simulink library "ammclib_bam_s32k11x"  (Simulink 9.0)
settings: Solver=ode45  StartTime=0.0  StopTime=10.0  RelTol=1e-3
undefined symbols (not defined in the file): f16A1, f16A2, f16B0, f16B1, f16B2, f16C1, f16CC1, f16CC1sc, f16CC1sc_D, f16CC1sc_Q, f16CC1scD, f16CC1scQ, f16CC2, f16CC2sc, f16CC2sc_D, f16CC2sc_Q, f16CC2scD, f16CC2scQ, f16DerivGain, f16EGain, f16FiltCoef, f16HystOff, f16HystOn, f16IGain, f16IntegGain, f16IntegGainFW, f16IntegGainQ, f16Kd, f16Kq, f16Limit, f16LowerLim, f16LowerLimit_D, f16LowerLimit_Q, f16ModIndex, f16OutValOff, f16OutValOn, f16PropGain, f16PropGainFW, f16PropGainQ, f16RampDown, f16RampUp, f16UGain, f16UpperLim, f16UpperLimit, f16UpperLimit_D, f16UpperLimit_Q, f16WIGain, f32A1, f32A2, f32B0, f32B1, f32B2, f32C1, f32CC1, f32CC1sc, f32CC1sc_D, f32CC1sc_Q, f32CC1scD, f32CC1scQ, f32CC2 ... (+71)
(part 7 of 7)

== system ammclib_bam_s32k11x/MLIB/bam_f32/MLIB_SubSat_F32 ==
  note: ---------------------------------------------------------------------------------------------------------------------------------------------------------------------------------------------------
  f32In1 : Inport
  f32In2 : Inport  Port=2
  MLIB_SubSat_SF : S-Function  FunctionName=MLIB_SubSat_SF_F32  SFunctionDeploymentMode=off  EnableBusSupport=off
  copyright : Subsystem
      mask Display:
      | text(10,90,'FILE:');text(10,75,'DESRIPTION:')
      | text(10,60,'COPYRIGHT:')
      | text(10,45,'VERSION:')
      | text(10,30,'DATE:')
  copyright2 : Subsystem
      mask Display:
      | text(10,90,'MLIB_SubSat_BAM_F32.mdl');text(10,75,'Saturated sum of two input values.');text(10,60,'NXP')
      | text(10,45,'0.1');text(10,30,'20-Jan-2012');
  logo : Subsystem
      mask Display: image(imread('logo.jpg'))
  f32Out : Outport
  wires:
  MLIB_SubSat_SF/1 -> f32Out/1
  f32In2/1 -> MLIB_SubSat_SF/2
  f32In1/1 -> MLIB_SubSat_SF/1

== system ammclib_bam_s32k11x/MLIB/bam_f32/MLIB_Sub_F32 ==
  note: ---------------------------------------------------------------------------------------------------------------------------------------------------------------------------------------------------
  f32In1 : Inport
  f32In2 : Inport  Port=2
  MLIB_Sub_SF : S-Function  FunctionName=MLIB_Sub_SF_F32  SFunctionDeploymentMode=off  EnableBusSupport=off
  copyright : Subsystem
      mask Display:
      | text(10,90,'FILE:');text(10,75,'DESRIPTION:')
      | text(10,60,'COPYRIGHT:')
      | text(10,45,'VERSION:')
      | text(10,30,'DATE:')
  copyright2 : Subsystem
      mask Display:
      | text(10,90,'MLIB_Sub_BAM_F32.mdl');text(10,75,'Sum of two input values.');text(10,60,'NXP')
      | text(10,45,'0.1');text(10,30,'18-Jul-2011');
  logo : Subsystem
      mask Display: image(imread('logo.jpg'))
  f32Out : Outport
  wires:
  MLIB_Sub_SF/1 -> f32Out/1
  f32In2/1 -> MLIB_Sub_SF/2
  f32In1/1 -> MLIB_Sub_SF/1

== system ammclib_bam_s32k11x/MLIB/bam_f32/MLIB_VMac_F32 ==
  note: ---------------------------------------------------------------------------------------------------------------------------------------------------------------------------------------------------
  f32In1 : Inport
  f32In2 : Inport  Port=2
  f32In3 : Inport  Port=3
  f32In4 : Inport  Port=4
  MLIB_VMac_SF : S-Function  FunctionName=MLIB_VMac_SF_F32  SFunctionDeploymentMode=off  EnableBusSupport=off
  copyright : Subsystem
      mask Display:
      | text(10,90,'FILE:');text(10,75,'DESRIPTION:')
      | text(10,60,'COPYRIGHT:')
      | text(10,45,'VERSION:')
      | text(10,30,'DATE:')
  copyright2 : Subsystem
      mask Display:
      | text(10,90,'MLIB_VMac_BAM_F32.mdl');text(10,75,'Vector multiply accumulate.');text(10,60,'Freescale')
      | text(10,45,'0.1');text(10,30,'25-Aug-2011');
  logo : Subsystem
      mask Display: image(imread('logo.jpg'))
  f32Out : Outport
  wires:
  MLIB_VMac_SF/1 -> f32Out/1
  f32In4/1 -> MLIB_VMac_SF/4
  f32In3/1 -> MLIB_VMac_SF/3
  f32In2/1 -> MLIB_VMac_SF/2
  f32In1/1 -> MLIB_VMac_SF/1

== system ammclib_bam_s32k11x/MLIB/bam_f32f16f16/MLIB_MacSat_F32F16F16 ==
  note: ---------------------------------------------------------------------------------------------------------------------------------------------------------------------------------------------------
  f32In1 : Inport
  f16In2 : Inport  Port=2
  f16In3 : Inport  Port=3
  MLIB_MacSat_SF : S-Function  FunctionName=MLIB_MacSat_SF_F32F16F16  SFunctionDeploymentMode=off  EnableBusSupport=off
  copyright : Subsystem
      mask Display:
      | text(10,90,'FILE:');text(10,75,'DESRIPTION:')
      | text(10,60,'COPYRIGHT:')
      | text(10,45,'VERSION:')
      | text(10,30,'DATE:')
  copyright2 : Subsystem
      mask Display:
      | text(10,90,'MLIB_MacSat_BAM_F32F16F16.mdl');text(10,75,'Multiplication of second and third input value and adding of first input value, staturated if necessary.');text(10,60,'NXP')
      | text(10,45,'0.1');text(10,30,'22-Aug-2011');
  logo : Subsystem
      mask Display: image(imread('logo.jpg'))
  f32Out : Outport
  wires:
  MLIB_MacSat_SF/1 -> f32Out/1
  f16In3/1 -> MLIB_MacSat_SF/3
  f16In2/1 -> MLIB_MacSat_SF/2
  f32In1/1 -> MLIB_MacSat_SF/1

== system ammclib_bam_s32k11x/MLIB/bam_f32f16f16/MLIB_Mac_F32F16F16 ==
  note: ---------------------------------------------------------------------------------------------------------------------------------------------------------------------------------------------------
  f32In1 : Inport
  f16In2 : Inport  Port=2
  f16In3 : Inport  Port=3
  MLIB_Mac_SF : S-Function  FunctionName=MLIB_Mac_SF_F32F16F16  SFunctionDeploymentMode=off  EnableBusSupport=off
  copyright : Subsystem
      mask Display:
      | text(10,90,'FILE:');text(10,75,'DESRIPTION:')
      | text(10,60,'COPYRIGHT:')
      | text(10,45,'VERSION:')
      | text(10,30,'DATE:')
  copyright2 : Subsystem
      mask Display:
      | text(10,90,'MLIB_Mac_BAM_F32F16F16.mdl');text(10,75,'Sum of two input values.');text(10,60,'Freescale')
      | text(10,45,'0.1');text(10,30,'18-Jul-2011');
  logo : Subsystem
      mask Display: image(imread('logo.jpg'))
  f32Out : Outport
  wires:
  MLIB_Mac_SF/1 -> f32Out/1
  f16In3/1 -> MLIB_Mac_SF/3
  f16In2/1 -> MLIB_Mac_SF/2
  f32In1/1 -> MLIB_Mac_SF/1

== system ammclib_bam_s32k11x/MLIB/bam_f32f16f16/MLIB_Mnac_F32F16F16 ==
  note: ---------------------------------------------------------------------------------------------------------------------------------------------------------------------------------------------------
  f32In1 : Inport
  f16In2 : Inport  Port=2
  f16In3 : Inport  Port=3
  MLIB_Mnac_SF : S-Function  FunctionName=MLIB_Mnac_SF_F32F16F16  SFunctionDeploymentMode=off  EnableBusSupport=off
  copyright : Subsystem
      mask Display:
      | text(10,90,'FILE:');text(10,75,'DESRIPTION:')
      | text(10,60,'COPYRIGHT:')
      | text(10,45,'VERSION:')
      | text(10,30,'DATE:')
  copyright2 : Subsystem
      mask Display:
      | text(10,90,'MLIB_Mnac_BAM_F32F16F16.mdl');text(10,75,'Multiply-negative-accumulate.');text(10,60,'NXP')
      | text(10,45,'1.0');text(10,30,'27-Mar-2015');
  logo : Subsystem
      mask Display: image(imread('logo.jpg'))
  f32Out : Outport
  wires:
  MLIB_Mnac_SF/1 -> f32Out/1
  f16In3/1 -> MLIB_Mnac_SF/3
  f16In2/1 -> MLIB_Mnac_SF/2
  f32In1/1 -> MLIB_Mnac_SF/1

== system ammclib_bam_s32k11x/MLIB/bam_f32f16f16/MLIB_Msu_F32F16F16 ==
  note: ---------------------------------------------------------------------------------------------------------------------------------------------------------------------------------------------------
  f32In1 : Inport
  f16In2 : Inport  Port=2
  f16In3 : Inport  Port=3
  MLIB_Msu_SF : S-Function  FunctionName=MLIB_Msu_SF_F32F16F16  SFunctionDeploymentMode=off  EnableBusSupport=off
  copyright : Subsystem
      mask Display:
      | text(10,90,'FILE:');text(10,75,'DESRIPTION:')
      | text(10,60,'COPYRIGHT:')
      | text(10,45,'VERSION:')
      | text(10,30,'DATE:')
  copyright2 : Subsystem
      mask Display:
      | text(10,90,'MLIB_Msu_BAM_F32F16F16.mdl');text(10,75,'Multiply-subtract-from.');text(10,60,'Freescale')
      | text(10,45,'1.0');text(10,30,'27-Mar-2015');
  logo : Subsystem
      mask Display: image(imread('logo.jpg'))
  f32Out : Outport
  wires:
  MLIB_Msu_SF/1 -> f32Out/1
  f16In3/1 -> MLIB_Msu_SF/3
  f16In2/1 -> MLIB_Msu_SF/2
  f32In1/1 -> MLIB_Msu_SF/1

== system ammclib_bam_s32k11x/MLIB/bam_f32f16f16/MLIB_MulSat_F32F16F16 ==
  note: ---------------------------------------------------------------------------------------------------------------------------------------------------------------------------------------------------
  f16In1 : Inport
  f16In2 : Inport  Port=2
  MLIB_MulSat_SF : S-Function  FunctionName=MLIB_MulSat_SF_F32F16F16  SFunctionDeploymentMode=off  EnableBusSupport=off
  copyright : Subsystem
      mask Display:
      | text(10,90,'FILE:');text(10,75,'DESRIPTION:')
      | text(10,60,'COPYRIGHT:')
      | text(10,45,'VERSION:')
      | text(10,30,'DATE:')
  copyright2 : Subsystem
      mask Display:
      | text(10,90,'MLIB_MulSat_BAM_F32F16F16.mdl');text(10,75,'Saturated sum of two input values.');text(10,60,'NXP')
      | text(10,45,'0.1');text(10,30,'01-Aug-2011');
  logo : Subsystem
      mask Display: image(imread('logo.jpg'))
  f32Out : Outport
  wires:
  MLIB_MulSat_SF/1 -> f32Out/1
  f16In2/1 -> MLIB_MulSat_SF/2
  f16In1/1 -> MLIB_MulSat_SF/1

== system ammclib_bam_s32k11x/MLIB/bam_f32f16f16/MLIB_Mul_F32F16F16 ==
  note: ---------------------------------------------------------------------------------------------------------------------------------------------------------------------------------------------------
  f16In1 : Inport
  f16In2 : Inport  Port=2
  MLIB_Mul_SF : S-Function  FunctionName=MLIB_Mul_SF_F32F16F16  SFunctionDeploymentMode=off  EnableBusSupport=off
  copyright : Subsystem
      mask Display:
      | text(10,90,'FILE:');text(10,75,'DESRIPTION:')
      | text(10,60,'COPYRIGHT:')
      | text(10,45,'VERSION:')
      | text(10,30,'DATE:')
  copyright2 : Subsystem
      mask Display:
      | text(10,90,'MLIB_Mul_BAM_F32F16F16.mdl');text(10,75,'Sum of two input values.');text(10,60,'Freescale')
      | text(10,45,'0.1');text(10,30,'26-Jul-2011');
  logo : Subsystem
      mask Display: image(imread('logo.jpg'))
  f32Out : Outport
  wires:
  MLIB_Mul_SF/1 -> f32Out/1
  f16In2/1 -> MLIB_Mul_SF/2
  f16In1/1 -> MLIB_Mul_SF/1

== system ammclib_bam_s32k11x/MLIB/bam_f32f16f16/MLIB_VMac_F32F16F16 ==
  note: ---------------------------------------------------------------------------------------------------------------------------------------------------------------------------------------------------
  f16In1 : Inport
  f16In2 : Inport  Port=2
  f16In3 : Inport  Port=3
  f16In4 : Inport  Port=4
  MLIB_VMac_SF : S-Function  FunctionName=MLIB_VMac_SF_F32F16F16  SFunctionDeploymentMode=off  EnableBusSupport=off
  copyright : Subsystem
      mask Display:
      | text(10,90,'FILE:');text(10,75,'DESRIPTION:')
      | text(10,60,'COPYRIGHT:')
      | text(10,45,'VERSION:')
      | text(10,30,'DATE:')
  copyright2 : Subsystem
      mask Display:
      | text(10,90,'MLIB_VMac_BAM_F32F16F16.mdl');text(10,75,'Vector multiply accumulate.');text(10,60,'Freescale')
      | text(10,45,'0.1');text(10,30,'25-Aug-2011');
  logo : Subsystem
      mask Display: image(imread('logo.jpg'))
  f32Out : Outport
  wires:
  MLIB_VMac_SF/1 -> f32Out/1
  f16In4/1 -> MLIB_VMac_SF/4
  f16In3/1 -> MLIB_VMac_SF/3
  f16In2/1 -> MLIB_VMac_SF/2
  f16In1/1 -> MLIB_VMac_SF/1

== system ammclib_bam_s32k11x/AMCLIB/bam_f16/AMCLIB_BemfObsrvDQ_F16/copyright ==

== system ammclib_bam_s32k11x/AMCLIB/bam_f16/AMCLIB_BemfObsrvDQ_F16/copyright2 ==

== system ammclib_bam_s32k11x/AMCLIB/bam_f16/AMCLIB_BemfObsrvDQ_F16/logo ==

== system ammclib_bam_s32k11x/AMCLIB/bam_f16/AMCLIB_CurrentLoop_F16/copyright ==

== system ammclib_bam_s32k11x/AMCLIB/bam_f16/AMCLIB_CurrentLoop_F16/copyright2 ==

== system ammclib_bam_s32k11x/AMCLIB/bam_f16/AMCLIB_CurrentLoop_F16/logo ==

== system ammclib_bam_s32k11x/AMCLIB/bam_f16/AMCLIB_FWSpeedLoop_F16/copyright ==

== system ammclib_bam_s32k11x/AMCLIB/bam_f16/AMCLIB_FWSpeedLoop_F16/copyright2 ==

== system ammclib_bam_s32k11x/AMCLIB/bam_f16/AMCLIB_FWSpeedLoop_F16/logo ==

== system ammclib_bam_s32k11x/AMCLIB/bam_f16/AMCLIB_FW_F16/copyright ==

== system ammclib_bam_s32k11x/AMCLIB/bam_f16/AMCLIB_FW_F16/copyright2 ==

== system ammclib_bam_s32k11x/AMCLIB/bam_f16/AMCLIB_FW_F16/logo ==

== system ammclib_bam_s32k11x/AMCLIB/bam_f16/AMCLIB_SpeedLoop_F16/copyright ==

== system ammclib_bam_s32k11x/AMCLIB/bam_f16/AMCLIB_SpeedLoop_F16/copyright2 ==

== system ammclib_bam_s32k11x/AMCLIB/bam_f16/AMCLIB_SpeedLoop_F16/logo ==

== system ammclib_bam_s32k11x/AMCLIB/bam_f16/AMCLIB_TrackObsrv_F16/copyright ==

== system ammclib_bam_s32k11x/AMCLIB/bam_f16/AMCLIB_TrackObsrv_F16/copyright2 ==

== system ammclib_bam_s32k11x/AMCLIB/bam_f16/AMCLIB_TrackObsrv_F16/logo ==

== system ammclib_bam_s32k11x/AMCLIB/bam_f32/AMCLIB_BemfObsrvDQ_F32/copyright ==

== system ammclib_bam_s32k11x/AMCLIB/bam_f32/AMCLIB_BemfObsrvDQ_F32/copyright2 ==

== system ammclib_bam_s32k11x/AMCLIB/bam_f32/AMCLIB_BemfObsrvDQ_F32/logo ==

== system ammclib_bam_s32k11x/AMCLIB/bam_f32/AMCLIB_CurrentLoop_F32/copyright ==

== system ammclib_bam_s32k11x/AMCLIB/bam_f32/AMCLIB_CurrentLoop_F32/copyright2 ==

== system ammclib_bam_s32k11x/AMCLIB/bam_f32/AMCLIB_CurrentLoop_F32/logo ==

== system ammclib_bam_s32k11x/AMCLIB/bam_f32/AMCLIB_FWSpeedLoop_F32/copyright ==

== system ammclib_bam_s32k11x/AMCLIB/bam_f32/AMCLIB_FWSpeedLoop_F32/copyright2 ==

== system ammclib_bam_s32k11x/AMCLIB/bam_f32/AMCLIB_FWSpeedLoop_F32/logo ==

== system ammclib_bam_s32k11x/AMCLIB/bam_f32/AMCLIB_FW_F32/copyright ==

== system ammclib_bam_s32k11x/AMCLIB/bam_f32/AMCLIB_FW_F32/copyright2 ==

== system ammclib_bam_s32k11x/AMCLIB/bam_f32/AMCLIB_FW_F32/logo ==

== system ammclib_bam_s32k11x/AMCLIB/bam_f32/AMCLIB_SpeedLoop_F32/copyright ==

== system ammclib_bam_s32k11x/AMCLIB/bam_f32/AMCLIB_SpeedLoop_F32/copyright2 ==

== system ammclib_bam_s32k11x/AMCLIB/bam_f32/AMCLIB_SpeedLoop_F32/logo ==

== system ammclib_bam_s32k11x/AMCLIB/bam_f32/AMCLIB_TrackObsrv_F32/copyright ==

== system ammclib_bam_s32k11x/AMCLIB/bam_f32/AMCLIB_TrackObsrv_F32/copyright2 ==

== system ammclib_bam_s32k11x/AMCLIB/bam_f32/AMCLIB_TrackObsrv_F32/logo ==

== system ammclib_bam_s32k11x/GDFLIB/bam_f16/GDFLIB_FilterFIR_F16/copyright ==

== system ammclib_bam_s32k11x/GDFLIB/bam_f16/GDFLIB_FilterFIR_F16/copyright2 ==

== system ammclib_bam_s32k11x/GDFLIB/bam_f16/GDFLIB_FilterFIR_F16/logo ==

== system ammclib_bam_s32k11x/GDFLIB/bam_f16/GDFLIB_FilterIIR1_F16/copyright ==

== system ammclib_bam_s32k11x/GDFLIB/bam_f16/GDFLIB_FilterIIR1_F16/copyright2 ==

== system ammclib_bam_s32k11x/GDFLIB/bam_f16/GDFLIB_FilterIIR1_F16/logo ==

== system ammclib_bam_s32k11x/GDFLIB/bam_f16/GDFLIB_FilterIIR2_F16/copyright ==

== system ammclib_bam_s32k11x/GDFLIB/bam_f16/GDFLIB_FilterIIR2_F16/copyright2 ==

== system ammclib_bam_s32k11x/GDFLIB/bam_f16/GDFLIB_FilterIIR2_F16/logo ==

== system ammclib_bam_s32k11x/GDFLIB/bam_f16/GDFLIB_FilterMA_F16/copyright ==

== system ammclib_bam_s32k11x/GDFLIB/bam_f16/GDFLIB_FilterMA_F16/copyright2 ==

== system ammclib_bam_s32k11x/GDFLIB/bam_f16/GDFLIB_FilterMA_F16/logo ==

== system ammclib_bam_s32k11x/GDFLIB/bam_f32/GDFLIB_FilterFIR_F32/copyright ==

== system ammclib_bam_s32k11x/GDFLIB/bam_f32/GDFLIB_FilterFIR_F32/copyright2 ==

== system ammclib_bam_s32k11x/GDFLIB/bam_f32/GDFLIB_FilterFIR_F32/logo ==

== system ammclib_bam_s32k11x/GDFLIB/bam_f32/GDFLIB_FilterIIR1_F32/copyright ==

== system ammclib_bam_s32k11x/GDFLIB/bam_f32/GDFLIB_FilterIIR1_F32/copyright2 ==

== system ammclib_bam_s32k11x/GDFLIB/bam_f32/GDFLIB_FilterIIR1_F32/logo ==

== system ammclib_bam_s32k11x/GDFLIB/bam_f32/GDFLIB_FilterIIR2_F32/copyright ==

== system ammclib_bam_s32k11x/GDFLIB/bam_f32/GDFLIB_FilterIIR2_F32/copyright2 ==

== system ammclib_bam_s32k11x/GDFLIB/bam_f32/GDFLIB_FilterIIR2_F32/logo ==

== system ammclib_bam_s32k11x/GDFLIB/bam_f32/GDFLIB_FilterMA_F32/copyright ==

== system ammclib_bam_s32k11x/GDFLIB/bam_f32/GDFLIB_FilterMA_F32/copyright2 ==

== system ammclib_bam_s32k11x/GDFLIB/bam_f32/GDFLIB_FilterMA_F32/logo ==

== system ammclib_bam_s32k11x/GFLIB/bam_f16/GFLIB_Acos_F16/copyright ==

== system ammclib_bam_s32k11x/GFLIB/bam_f16/GFLIB_Acos_F16/copyright2 ==

== system ammclib_bam_s32k11x/GFLIB/bam_f16/GFLIB_Acos_F16/logo ==

== system ammclib_bam_s32k11x/GFLIB/bam_f16/GFLIB_Asin_F16/copyright ==

== system ammclib_bam_s32k11x/GFLIB/bam_f16/GFLIB_Asin_F16/copyright2 ==

== system ammclib_bam_s32k11x/GFLIB/bam_f16/GFLIB_Asin_F16/logo ==

== system ammclib_bam_s32k11x/GFLIB/bam_f16/GFLIB_AtanYXShifted_F16/copyright ==

== system ammclib_bam_s32k11x/GFLIB/bam_f16/GFLIB_AtanYXShifted_F16/copyright2 ==

== system ammclib_bam_s32k11x/GFLIB/bam_f16/GFLIB_AtanYXShifted_F16/logo ==

== system ammclib_bam_s32k11x/GFLIB/bam_f16/GFLIB_AtanYX_F16/copyright ==

== system ammclib_bam_s32k11x/GFLIB/bam_f16/GFLIB_AtanYX_F16/copyright2 ==

== system ammclib_bam_s32k11x/GFLIB/bam_f16/GFLIB_AtanYX_F16/logo ==

== system ammclib_bam_s32k11x/GFLIB/bam_f16/GFLIB_Atan_F16/copyright ==

== system ammclib_bam_s32k11x/GFLIB/bam_f16/GFLIB_Atan_F16/copyright2 ==

== system ammclib_bam_s32k11x/GFLIB/bam_f16/GFLIB_Atan_F16/logo ==

== system ammclib_bam_s32k11x/GFLIB/bam_f16/GFLIB_ControllerPIDpAW_F16/copyright ==

== system ammclib_bam_s32k11x/GFLIB/bam_f16/GFLIB_ControllerPIDpAW_F16/copyright2 ==

== system ammclib_bam_s32k11x/GFLIB/bam_f16/GFLIB_ControllerPIDpAW_F16/logo ==

== system ammclib_bam_s32k11x/GFLIB/bam_f16/GFLIB_ControllerPIpAW_F16/copyright ==

== system ammclib_bam_s32k11x/GFLIB/bam_f16/GFLIB_ControllerPIpAW_F16/copyright2 ==

== system ammclib_bam_s32k11x/GFLIB/bam_f16/GFLIB_ControllerPIpAW_F16/logo ==

== system ammclib_bam_s32k11x/GFLIB/bam_f16/GFLIB_ControllerPIp_F16/copyright ==

== system ammclib_bam_s32k11x/GFLIB/bam_f16/GFLIB_ControllerPIp_F16/copyright2 ==

== system ammclib_bam_s32k11x/GFLIB/bam_f16/GFLIB_ControllerPIp_F16/logo ==

== system ammclib_bam_s32k11x/GFLIB/bam_f16/GFLIB_ControllerPIrAW_F16/copyright ==

== system ammclib_bam_s32k11x/GFLIB/bam_f16/GFLIB_ControllerPIrAW_F16/copyright2 ==

== system ammclib_bam_s32k11x/GFLIB/bam_f16/GFLIB_ControllerPIrAW_F16/logo ==

== system ammclib_bam_s32k11x/GFLIB/bam_f16/GFLIB_ControllerPIr_F16/copyright ==

== system ammclib_bam_s32k11x/GFLIB/bam_f16/GFLIB_ControllerPIr_F16/copyright2 ==

== system ammclib_bam_s32k11x/GFLIB/bam_f16/GFLIB_ControllerPIr_F16/logo ==

== system ammclib_bam_s32k11x/GFLIB/bam_f16/GFLIB_Cos_F16/copyright ==

== system ammclib_bam_s32k11x/GFLIB/bam_f16/GFLIB_Cos_F16/copyright2 ==

== system ammclib_bam_s32k11x/GFLIB/bam_f16/GFLIB_Cos_F16/logo ==

== system ammclib_bam_s32k11x/GFLIB/bam_f16/GFLIB_Hyst_F16/copyright ==

== system ammclib_bam_s32k11x/GFLIB/bam_f16/GFLIB_Hyst_F16/copyright2 ==

== system ammclib_bam_s32k11x/GFLIB/bam_f16/GFLIB_Hyst_F16/logo ==

== system ammclib_bam_s32k11x/GFLIB/bam_f16/GFLIB_IntegratorTR_F16/copyright ==

== system ammclib_bam_s32k11x/GFLIB/bam_f16/GFLIB_IntegratorTR_F16/copyright2 ==

== system ammclib_bam_s32k11x/GFLIB/bam_f16/GFLIB_IntegratorTR_F16/logo ==

== system ammclib_bam_s32k11x/GFLIB/bam_f16/GFLIB_Limit_F16/copyright ==

== system ammclib_bam_s32k11x/GFLIB/bam_f16/GFLIB_Limit_F16/copyright2 ==

== system ammclib_bam_s32k11x/GFLIB/bam_f16/GFLIB_Limit_F16/logo ==

== system ammclib_bam_s32k11x/GFLIB/bam_f16/GFLIB_LowerLimit_F16/copyright ==

== system ammclib_bam_s32k11x/GFLIB/bam_f16/GFLIB_LowerLimit_F16/copyright2 ==

== system ammclib_bam_s32k11x/GFLIB/bam_f16/GFLIB_LowerLimit_F16/logo ==

== system ammclib_bam_s32k11x/GFLIB/bam_f16/GFLIB_Lut1D_F16/copyright ==

== system ammclib_bam_s32k11x/GFLIB/bam_f16/GFLIB_Lut1D_F16/copyright2 ==

== system ammclib_bam_s32k11x/GFLIB/bam_f16/GFLIB_Lut1D_F16/logo ==

== system ammclib_bam_s32k11x/GFLIB/bam_f16/GFLIB_Lut2D_F16/copyright ==

== system ammclib_bam_s32k11x/GFLIB/bam_f16/GFLIB_Lut2D_F16/copyright2 ==

== system ammclib_bam_s32k11x/GFLIB/bam_f16/GFLIB_Lut2D_F16/logo ==

== system ammclib_bam_s32k11x/GFLIB/bam_f16/GFLIB_Ramp_F16/copyright ==

== system ammclib_bam_s32k11x/GFLIB/bam_f16/GFLIB_Ramp_F16/copyright2 ==

== system ammclib_bam_s32k11x/GFLIB/bam_f16/GFLIB_Ramp_F16/logo ==

== system ammclib_bam_s32k11x/GFLIB/bam_f16/GFLIB_Sign_F16/copyright ==

== system ammclib_bam_s32k11x/GFLIB/bam_f16/GFLIB_Sign_F16/copyright2 ==

== system ammclib_bam_s32k11x/GFLIB/bam_f16/GFLIB_Sign_F16/logo ==

== system ammclib_bam_s32k11x/GFLIB/bam_f16/GFLIB_SinCos_F16/copyright ==

== system ammclib_bam_s32k11x/GFLIB/bam_f16/GFLIB_SinCos_F16/copyright2 ==

== system ammclib_bam_s32k11x/GFLIB/bam_f16/GFLIB_SinCos_F16/logo ==

== system ammclib_bam_s32k11x/GFLIB/bam_f16/GFLIB_Sin_F16/copyright ==

== system ammclib_bam_s32k11x/GFLIB/bam_f16/GFLIB_Sin_F16/copyright2 ==

== system ammclib_bam_s32k11x/GFLIB/bam_f16/GFLIB_Sin_F16/logo ==

== system ammclib_bam_s32k11x/GFLIB/bam_f16/GFLIB_Sqrt_F16/copyright ==

== system ammclib_bam_s32k11x/GFLIB/bam_f16/GFLIB_Sqrt_F16/copyright2 ==

== system ammclib_bam_s32k11x/GFLIB/bam_f16/GFLIB_Sqrt_F16/logo ==

== system ammclib_bam_s32k11x/GFLIB/bam_f16/GFLIB_Tan_F16/copyright ==

== system ammclib_bam_s32k11x/GFLIB/bam_f16/GFLIB_Tan_F16/copyright2 ==

== system ammclib_bam_s32k11x/GFLIB/bam_f16/GFLIB_Tan_F16/logo ==

== system ammclib_bam_s32k11x/GFLIB/bam_f16/GFLIB_UpperLimit_F16/copyright ==

== system ammclib_bam_s32k11x/GFLIB/bam_f16/GFLIB_UpperLimit_F16/copyright2 ==

== system ammclib_bam_s32k11x/GFLIB/bam_f16/GFLIB_UpperLimit_F16/logo ==

== system ammclib_bam_s32k11x/GFLIB/bam_f16/GFLIB_VMin_F16/copyright ==

== system ammclib_bam_s32k11x/GFLIB/bam_f16/GFLIB_VMin_F16/copyright2 ==

== system ammclib_bam_s32k11x/GFLIB/bam_f16/GFLIB_VMin_F16/logo ==

== system ammclib_bam_s32k11x/GFLIB/bam_f16/GFLIB_VectorLimit_F16/copyright ==

== system ammclib_bam_s32k11x/GFLIB/bam_f16/GFLIB_VectorLimit_F16/copyright2 ==

== system ammclib_bam_s32k11x/GFLIB/bam_f16/GFLIB_VectorLimit_F16/logo ==

== system ammclib_bam_s32k11x/GFLIB/bam_f32/GFLIB_Acos_F32/copyright ==

== system ammclib_bam_s32k11x/GFLIB/bam_f32/GFLIB_Acos_F32/copyright2 ==

== system ammclib_bam_s32k11x/GFLIB/bam_f32/GFLIB_Acos_F32/logo ==

== system ammclib_bam_s32k11x/GFLIB/bam_f32/GFLIB_Asin_F32/copyright ==

== system ammclib_bam_s32k11x/GFLIB/bam_f32/GFLIB_Asin_F32/copyright2 ==

== system ammclib_bam_s32k11x/GFLIB/bam_f32/GFLIB_Asin_F32/logo ==

== system ammclib_bam_s32k11x/GFLIB/bam_f32/GFLIB_AtanYXShifted_F32/copyright ==

== system ammclib_bam_s32k11x/GFLIB/bam_f32/GFLIB_AtanYXShifted_F32/copyright2 ==

== system ammclib_bam_s32k11x/GFLIB/bam_f32/GFLIB_AtanYXShifted_F32/logo ==

== system ammclib_bam_s32k11x/GFLIB/bam_f32/GFLIB_AtanYX_F32/copyright ==

== system ammclib_bam_s32k11x/GFLIB/bam_f32/GFLIB_AtanYX_F32/copyright2 ==

== system ammclib_bam_s32k11x/GFLIB/bam_f32/GFLIB_AtanYX_F32/logo ==

== system ammclib_bam_s32k11x/GFLIB/bam_f32/GFLIB_Atan_F32/copyright ==

== system ammclib_bam_s32k11x/GFLIB/bam_f32/GFLIB_Atan_F32/copyright2 ==

== system ammclib_bam_s32k11x/GFLIB/bam_f32/GFLIB_Atan_F32/logo ==

== system ammclib_bam_s32k11x/GFLIB/bam_f32/GFLIB_ControllerPIDpAW_F32/copyright ==

== system ammclib_bam_s32k11x/GFLIB/bam_f32/GFLIB_ControllerPIDpAW_F32/copyright2 ==

== system ammclib_bam_s32k11x/GFLIB/bam_f32/GFLIB_ControllerPIDpAW_F32/logo ==

== system ammclib_bam_s32k11x/GFLIB/bam_f32/GFLIB_ControllerPIpAW_F32/copyright ==

== system ammclib_bam_s32k11x/GFLIB/bam_f32/GFLIB_ControllerPIpAW_F32/copyright2 ==

== system ammclib_bam_s32k11x/GFLIB/bam_f32/GFLIB_ControllerPIpAW_F32/logo ==

== system ammclib_bam_s32k11x/GFLIB/bam_f32/GFLIB_ControllerPIp_F32/copyright ==

== system ammclib_bam_s32k11x/GFLIB/bam_f32/GFLIB_ControllerPIp_F32/copyright2 ==

== system ammclib_bam_s32k11x/GFLIB/bam_f32/GFLIB_ControllerPIp_F32/logo ==

== system ammclib_bam_s32k11x/GFLIB/bam_f32/GFLIB_ControllerPIrAW_F32/copyright ==

== system ammclib_bam_s32k11x/GFLIB/bam_f32/GFLIB_ControllerPIrAW_F32/copyright2 ==

== system ammclib_bam_s32k11x/GFLIB/bam_f32/GFLIB_ControllerPIrAW_F32/logo ==

== system ammclib_bam_s32k11x/GFLIB/bam_f32/GFLIB_ControllerPIr_F32/copyright ==

== system ammclib_bam_s32k11x/GFLIB/bam_f32/GFLIB_ControllerPIr_F32/copyright2 ==

== system ammclib_bam_s32k11x/GFLIB/bam_f32/GFLIB_ControllerPIr_F32/logo ==

== system ammclib_bam_s32k11x/GFLIB/bam_f32/GFLIB_Cos_F32/copyright ==

== system ammclib_bam_s32k11x/GFLIB/bam_f32/GFLIB_Cos_F32/copyright2 ==

== system ammclib_bam_s32k11x/GFLIB/bam_f32/GFLIB_Cos_F32/logo ==

== system ammclib_bam_s32k11x/GFLIB/bam_f32/GFLIB_Hyst_F32/copyright ==

== system ammclib_bam_s32k11x/GFLIB/bam_f32/GFLIB_Hyst_F32/copyright2 ==

== system ammclib_bam_s32k11x/GFLIB/bam_f32/GFLIB_Hyst_F32/logo ==

== system ammclib_bam_s32k11x/GFLIB/bam_f32/GFLIB_IntegratorTR_F32/copyright ==

== system ammclib_bam_s32k11x/GFLIB/bam_f32/GFLIB_IntegratorTR_F32/copyright2 ==

== system ammclib_bam_s32k11x/GFLIB/bam_f32/GFLIB_IntegratorTR_F32/logo ==

== system ammclib_bam_s32k11x/GFLIB/bam_f32/GFLIB_Limit_F32/copyright ==

== system ammclib_bam_s32k11x/GFLIB/bam_f32/GFLIB_Limit_F32/copyright2 ==

== system ammclib_bam_s32k11x/GFLIB/bam_f32/GFLIB_Limit_F32/logo ==

== system ammclib_bam_s32k11x/GFLIB/bam_f32/GFLIB_LowerLimit_F32/copyright ==

== system ammclib_bam_s32k11x/GFLIB/bam_f32/GFLIB_LowerLimit_F32/copyright2 ==

== system ammclib_bam_s32k11x/GFLIB/bam_f32/GFLIB_LowerLimit_F32/logo ==

== system ammclib_bam_s32k11x/GFLIB/bam_f32/GFLIB_Lut1D_F32/copyright ==

== system ammclib_bam_s32k11x/GFLIB/bam_f32/GFLIB_Lut1D_F32/copyright2 ==

== system ammclib_bam_s32k11x/GFLIB/bam_f32/GFLIB_Lut1D_F32/logo ==

== system ammclib_bam_s32k11x/GFLIB/bam_f32/GFLIB_Lut2D_F32/copyright ==

== system ammclib_bam_s32k11x/GFLIB/bam_f32/GFLIB_Lut2D_F32/copyright2 ==

== system ammclib_bam_s32k11x/GFLIB/bam_f32/GFLIB_Lut2D_F32/logo ==

== system ammclib_bam_s32k11x/GFLIB/bam_f32/GFLIB_Ramp_F32/copyright ==

== system ammclib_bam_s32k11x/GFLIB/bam_f32/GFLIB_Ramp_F32/copyright2 ==

== system ammclib_bam_s32k11x/GFLIB/bam_f32/GFLIB_Ramp_F32/logo ==

== system ammclib_bam_s32k11x/GFLIB/bam_f32/GFLIB_Sign_F32/copyright ==

== system ammclib_bam_s32k11x/GFLIB/bam_f32/GFLIB_Sign_F32/copyright2 ==

== system ammclib_bam_s32k11x/GFLIB/bam_f32/GFLIB_Sign_F32/logo ==

== system ammclib_bam_s32k11x/GFLIB/bam_f32/GFLIB_SinCos_F32/copyright ==

== system ammclib_bam_s32k11x/GFLIB/bam_f32/GFLIB_SinCos_F32/copyright2 ==

== system ammclib_bam_s32k11x/GFLIB/bam_f32/GFLIB_SinCos_F32/logo ==

== system ammclib_bam_s32k11x/GFLIB/bam_f32/GFLIB_Sin_F32/copyright ==

== system ammclib_bam_s32k11x/GFLIB/bam_f32/GFLIB_Sin_F32/copyright2 ==

== system ammclib_bam_s32k11x/GFLIB/bam_f32/GFLIB_Sin_F32/logo ==

== system ammclib_bam_s32k11x/GFLIB/bam_f32/GFLIB_Sqrt_F32/copyright ==

== system ammclib_bam_s32k11x/GFLIB/bam_f32/GFLIB_Sqrt_F32/copyright2 ==

== system ammclib_bam_s32k11x/GFLIB/bam_f32/GFLIB_Sqrt_F32/logo ==

== system ammclib_bam_s32k11x/GFLIB/bam_f32/GFLIB_Tan_F32/copyright ==

== system ammclib_bam_s32k11x/GFLIB/bam_f32/GFLIB_Tan_F32/copyright2 ==

== system ammclib_bam_s32k11x/GFLIB/bam_f32/GFLIB_Tan_F32/logo ==

== system ammclib_bam_s32k11x/GFLIB/bam_f32/GFLIB_UpperLimit_F32/copyright ==

== system ammclib_bam_s32k11x/GFLIB/bam_f32/GFLIB_UpperLimit_F32/copyright2 ==

== system ammclib_bam_s32k11x/GFLIB/bam_f32/GFLIB_UpperLimit_F32/logo ==

== system ammclib_bam_s32k11x/GFLIB/bam_f32/GFLIB_VMin_F32/copyright ==

== system ammclib_bam_s32k11x/GFLIB/bam_f32/GFLIB_VMin_F32/copyright2 ==

== system ammclib_bam_s32k11x/GFLIB/bam_f32/GFLIB_VMin_F32/logo ==

== system ammclib_bam_s32k11x/GFLIB/bam_f32/GFLIB_VectorLimit_F32/copyright ==

== system ammclib_bam_s32k11x/GFLIB/bam_f32/GFLIB_VectorLimit_F32/copyright2 ==

== system ammclib_bam_s32k11x/GFLIB/bam_f32/GFLIB_VectorLimit_F32/logo ==

== system ammclib_bam_s32k11x/GMCLIB/bam_f16/GMCLIB_ClarkInv_F16/copyright ==

== system ammclib_bam_s32k11x/GMCLIB/bam_f16/GMCLIB_ClarkInv_F16/copyright2 ==

== system ammclib_bam_s32k11x/GMCLIB/bam_f16/GMCLIB_ClarkInv_F16/logo ==

== system ammclib_bam_s32k11x/GMCLIB/bam_f16/GMCLIB_Clark_F16/copyright ==

== system ammclib_bam_s32k11x/GMCLIB/bam_f16/GMCLIB_Clark_F16/copyright2 ==

== system ammclib_bam_s32k11x/GMCLIB/bam_f16/GMCLIB_Clark_F16/logo ==

== system ammclib_bam_s32k11x/GMCLIB/bam_f16/GMCLIB_DecouplingPMSM_F16/copyright ==

== system ammclib_bam_s32k11x/GMCLIB/bam_f16/GMCLIB_DecouplingPMSM_F16/copyright2 ==

== system ammclib_bam_s32k11x/GMCLIB/bam_f16/GMCLIB_DecouplingPMSM_F16/logo ==

== system ammclib_bam_s32k11x/GMCLIB/bam_f16/GMCLIB_ElimDcBusRip_F16/copyright ==

== system ammclib_bam_s32k11x/GMCLIB/bam_f16/GMCLIB_ElimDcBusRip_F16/copyright2 ==

== system ammclib_bam_s32k11x/GMCLIB/bam_f16/GMCLIB_ElimDcBusRip_F16/logo ==

== system ammclib_bam_s32k11x/GMCLIB/bam_f16/GMCLIB_ParkInv_F16/copyright ==

== system ammclib_bam_s32k11x/GMCLIB/bam_f16/GMCLIB_ParkInv_F16/copyright2 ==

== system ammclib_bam_s32k11x/GMCLIB/bam_f16/GMCLIB_ParkInv_F16/logo ==

== system ammclib_bam_s32k11x/GMCLIB/bam_f16/GMCLIB_Park_F16/copyright ==

== system ammclib_bam_s32k11x/GMCLIB/bam_f16/GMCLIB_Park_F16/copyright2 ==

== system ammclib_bam_s32k11x/GMCLIB/bam_f16/GMCLIB_Park_F16/logo ==

== system ammclib_bam_s32k11x/GMCLIB/bam_f16/GMCLIB_PwmIct_F16/copyright ==

== system ammclib_bam_s32k11x/GMCLIB/bam_f16/GMCLIB_PwmIct_F16/copyright2 ==

== system ammclib_bam_s32k11x/GMCLIB/bam_f16/GMCLIB_PwmIct_F16/logo ==

== system ammclib_bam_s32k11x/GMCLIB/bam_f16/GMCLIB_SvmStd_F16/copyright ==

== system ammclib_bam_s32k11x/GMCLIB/bam_f16/GMCLIB_SvmStd_F16/copyright2 ==

== system ammclib_bam_s32k11x/GMCLIB/bam_f16/GMCLIB_SvmStd_F16/logo ==

== system ammclib_bam_s32k11x/GMCLIB/bam_f16/GMCLIB_SvmU0n_F16/copyright ==

== system ammclib_bam_s32k11x/GMCLIB/bam_f16/GMCLIB_SvmU0n_F16/copyright2 ==

== system ammclib_bam_s32k11x/GMCLIB/bam_f16/GMCLIB_SvmU0n_F16/logo ==

== system ammclib_bam_s32k11x/GMCLIB/bam_f32/GMCLIB_ClarkInv_F32/copyright ==

== system ammclib_bam_s32k11x/GMCLIB/bam_f32/GMCLIB_ClarkInv_F32/copyright2 ==

== system ammclib_bam_s32k11x/GMCLIB/bam_f32/GMCLIB_ClarkInv_F32/logo ==

== system ammclib_bam_s32k11x/GMCLIB/bam_f32/GMCLIB_Clark_F32/copyright ==

== system ammclib_bam_s32k11x/GMCLIB/bam_f32/GMCLIB_Clark_F32/copyright2 ==

== system ammclib_bam_s32k11x/GMCLIB/bam_f32/GMCLIB_Clark_F32/logo ==

== system ammclib_bam_s32k11x/GMCLIB/bam_f32/GMCLIB_DecouplingPMSM_F32/copyright ==

== system ammclib_bam_s32k11x/GMCLIB/bam_f32/GMCLIB_DecouplingPMSM_F32/copyright2 ==

== system ammclib_bam_s32k11x/GMCLIB/bam_f32/GMCLIB_DecouplingPMSM_F32/logo ==

== system ammclib_bam_s32k11x/GMCLIB/bam_f32/GMCLIB_ElimDcBusRip_F32/copyright ==

== system ammclib_bam_s32k11x/GMCLIB/bam_f32/GMCLIB_ElimDcBusRip_F32/copyright2 ==

== system ammclib_bam_s32k11x/GMCLIB/bam_f32/GMCLIB_ElimDcBusRip_F32/logo ==

== system ammclib_bam_s32k11x/GMCLIB/bam_f32/GMCLIB_ParkInv_F32/copyright ==

== system ammclib_bam_s32k11x/GMCLIB/bam_f32/GMCLIB_ParkInv_F32/copyright2 ==

== system ammclib_bam_s32k11x/GMCLIB/bam_f32/GMCLIB_ParkInv_F32/logo ==

== system ammclib_bam_s32k11x/GMCLIB/bam_f32/GMCLIB_Park_F32/copyright ==

== system ammclib_bam_s32k11x/GMCLIB/bam_f32/GMCLIB_Park_F32/copyright2 ==

== system ammclib_bam_s32k11x/GMCLIB/bam_f32/GMCLIB_Park_F32/logo ==

== system ammclib_bam_s32k11x/GMCLIB/bam_f32/GMCLIB_PwmIct_F32/copyright ==

== system ammclib_bam_s32k11x/GMCLIB/bam_f32/GMCLIB_PwmIct_F32/copyright2 ==

== system ammclib_bam_s32k11x/GMCLIB/bam_f32/GMCLIB_PwmIct_F32/logo ==

== system ammclib_bam_s32k11x/GMCLIB/bam_f32/GMCLIB_SvmStd_F32/copyright ==

== system ammclib_bam_s32k11x/GMCLIB/bam_f32/GMCLIB_SvmStd_F32/copyright2 ==

== system ammclib_bam_s32k11x/GMCLIB/bam_f32/GMCLIB_SvmStd_F32/logo ==

== system ammclib_bam_s32k11x/GMCLIB/bam_f32/GMCLIB_SvmU0n_F32/copyright ==

== system ammclib_bam_s32k11x/GMCLIB/bam_f32/GMCLIB_SvmU0n_F32/copyright2 ==

== system ammclib_bam_s32k11x/GMCLIB/bam_f32/GMCLIB_SvmU0n_F32/logo ==

== system ammclib_bam_s32k11x/MLIB/bam_f16/MLIB_AbsSat_F16/copyright ==

== system ammclib_bam_s32k11x/MLIB/bam_f16/MLIB_AbsSat_F16/copyright2 ==

== system ammclib_bam_s32k11x/MLIB/bam_f16/MLIB_AbsSat_F16/logo ==

== system ammclib_bam_s32k11x/MLIB/bam_f16/MLIB_Abs_F16/copyright ==

== system ammclib_bam_s32k11x/MLIB/bam_f16/MLIB_Abs_F16/copyright2 ==

== system ammclib_bam_s32k11x/MLIB/bam_f16/MLIB_Abs_F16/logo ==

== system ammclib_bam_s32k11x/MLIB/bam_f16/MLIB_AddSat_F16/copyright ==

== system ammclib_bam_s32k11x/MLIB/bam_f16/MLIB_AddSat_F16/copyright2 ==

== system ammclib_bam_s32k11x/MLIB/bam_f16/MLIB_AddSat_F16/logo ==

== system ammclib_bam_s32k11x/MLIB/bam_f16/MLIB_Add_F16/copyright ==

== system ammclib_bam_s32k11x/MLIB/bam_f16/MLIB_Add_F16/copyright2 ==

== system ammclib_bam_s32k11x/MLIB/bam_f16/MLIB_Add_F16/logo ==

== system ammclib_bam_s32k11x/MLIB/bam_f16/MLIB_ConvertPU_F16F32/copyright ==

== system ammclib_bam_s32k11x/MLIB/bam_f16/MLIB_ConvertPU_F16F32/copyright2 ==

== system ammclib_bam_s32k11x/MLIB/bam_f16/MLIB_ConvertPU_F16F32/logo ==

== system ammclib_bam_s32k11x/MLIB/bam_f16/MLIB_Convert_F16F32/copyright ==

== system ammclib_bam_s32k11x/MLIB/bam_f16/MLIB_Convert_F16F32/copyright2 ==

== system ammclib_bam_s32k11x/MLIB/bam_f16/MLIB_Convert_F16F32/logo ==

== system ammclib_bam_s32k11x/MLIB/bam_f16/MLIB_DivSat_F16/copyright ==

== system ammclib_bam_s32k11x/MLIB/bam_f16/MLIB_DivSat_F16/copyright2 ==

== system ammclib_bam_s32k11x/MLIB/bam_f16/MLIB_DivSat_F16/logo ==

== system ammclib_bam_s32k11x/MLIB/bam_f16/MLIB_Div_F16/copyright ==

== system ammclib_bam_s32k11x/MLIB/bam_f16/MLIB_Div_F16/copyright2 ==

== system ammclib_bam_s32k11x/MLIB/bam_f16/MLIB_Div_F16/logo ==

== system ammclib_bam_s32k11x/MLIB/bam_f16/MLIB_MacSat_F16/copyright ==

== system ammclib_bam_s32k11x/MLIB/bam_f16/MLIB_MacSat_F16/copyright2 ==

== system ammclib_bam_s32k11x/MLIB/bam_f16/MLIB_MacSat_F16/logo ==

== system ammclib_bam_s32k11x/MLIB/bam_f16/MLIB_Mac_F16/copyright ==

== system ammclib_bam_s32k11x/MLIB/bam_f16/MLIB_Mac_F16/copyright2 ==

== system ammclib_bam_s32k11x/MLIB/bam_f16/MLIB_Mac_F16/logo ==

== system ammclib_bam_s32k11x/MLIB/bam_f16/MLIB_Mnac_F16/copyright ==

== system ammclib_bam_s32k11x/MLIB/bam_f16/MLIB_Mnac_F16/copyright2 ==

== system ammclib_bam_s32k11x/MLIB/bam_f16/MLIB_Mnac_F16/logo ==

== system ammclib_bam_s32k11x/MLIB/bam_f16/MLIB_Msu_F16/copyright ==

== system ammclib_bam_s32k11x/MLIB/bam_f16/MLIB_Msu_F16/copyright2 ==

== system ammclib_bam_s32k11x/MLIB/bam_f16/MLIB_Msu_F16/logo ==

== system ammclib_bam_s32k11x/MLIB/bam_f16/MLIB_MulSat_F16/copyright ==

== system ammclib_bam_s32k11x/MLIB/bam_f16/MLIB_MulSat_F16/copyright2 ==

== system ammclib_bam_s32k11x/MLIB/bam_f16/MLIB_MulSat_F16/logo ==

== system ammclib_bam_s32k11x/MLIB/bam_f16/MLIB_Mul_F16/copyright ==

== system ammclib_bam_s32k11x/MLIB/bam_f16/MLIB_Mul_F16/copyright2 ==

== system ammclib_bam_s32k11x/MLIB/bam_f16/MLIB_Mul_F16/logo ==

== system ammclib_bam_s32k11x/MLIB/bam_f16/MLIB_NegSat_F16/copyright ==

== system ammclib_bam_s32k11x/MLIB/bam_f16/MLIB_NegSat_F16/copyright2 ==

== system ammclib_bam_s32k11x/MLIB/bam_f16/MLIB_NegSat_F16/logo ==

== system ammclib_bam_s32k11x/MLIB/bam_f16/MLIB_Neg_F16/copyright ==

== system ammclib_bam_s32k11x/MLIB/bam_f16/MLIB_Neg_F16/copyright2 ==

== system ammclib_bam_s32k11x/MLIB/bam_f16/MLIB_Neg_F16/logo ==

== system ammclib_bam_s32k11x/MLIB/bam_f16/MLIB_Norm_F16/copyright ==

== system ammclib_bam_s32k11x/MLIB/bam_f16/MLIB_Norm_F16/copyright2 ==

== system ammclib_bam_s32k11x/MLIB/bam_f16/MLIB_Norm_F16/logo ==

== system ammclib_bam_s32k11x/MLIB/bam_f16/MLIB_RndSat_F16F32/copyright ==

== system ammclib_bam_s32k11x/MLIB/bam_f16/MLIB_RndSat_F16F32/copyright2 ==

== system ammclib_bam_s32k11x/MLIB/bam_f16/MLIB_RndSat_F16F32/logo ==

== system ammclib_bam_s32k11x/MLIB/bam_f16/MLIB_Round_F16/copyright ==

== system ammclib_bam_s32k11x/MLIB/bam_f16/MLIB_Round_F16/copyright2 ==

== system ammclib_bam_s32k11x/MLIB/bam_f16/MLIB_Round_F16/logo ==

== system ammclib_bam_s32k11x/MLIB/bam_f16/MLIB_ShBiSat_F16/copyright ==

== system ammclib_bam_s32k11x/MLIB/bam_f16/MLIB_ShBiSat_F16/copyright2 ==

== system ammclib_bam_s32k11x/MLIB/bam_f16/MLIB_ShBiSat_F16/logo ==

== system ammclib_bam_s32k11x/MLIB/bam_f16/MLIB_ShBi_F16/copyright ==

== system ammclib_bam_s32k11x/MLIB/bam_f16/MLIB_ShBi_F16/copyright2 ==

== system ammclib_bam_s32k11x/MLIB/bam_f16/MLIB_ShBi_F16/logo ==

== system ammclib_bam_s32k11x/MLIB/bam_f16/MLIB_ShLSat_F16/copyright ==

== system ammclib_bam_s32k11x/MLIB/bam_f16/MLIB_ShLSat_F16/copyright2 ==

== system ammclib_bam_s32k11x/MLIB/bam_f16/MLIB_ShLSat_F16/logo ==

== system ammclib_bam_s32k11x/MLIB/bam_f16/MLIB_ShL_F16/copyright ==

== system ammclib_bam_s32k11x/MLIB/bam_f16/MLIB_ShL_F16/copyright2 ==

== system ammclib_bam_s32k11x/MLIB/bam_f16/MLIB_ShL_F16/logo ==

== system ammclib_bam_s32k11x/MLIB/bam_f16/MLIB_ShR_F16/copyright ==

== system ammclib_bam_s32k11x/MLIB/bam_f16/MLIB_ShR_F16/copyright2 ==

== system ammclib_bam_s32k11x/MLIB/bam_f16/MLIB_ShR_F16/logo ==

== system ammclib_bam_s32k11x/MLIB/bam_f16/MLIB_SubSat_F16/copyright ==

== system ammclib_bam_s32k11x/MLIB/bam_f16/MLIB_SubSat_F16/copyright2 ==

== system ammclib_bam_s32k11x/MLIB/bam_f16/MLIB_SubSat_F16/logo ==

== system ammclib_bam_s32k11x/MLIB/bam_f16/MLIB_Sub_F16/copyright ==

== system ammclib_bam_s32k11x/MLIB/bam_f16/MLIB_Sub_F16/copyright2 ==

== system ammclib_bam_s32k11x/MLIB/bam_f16/MLIB_Sub_F16/logo ==

== system ammclib_bam_s32k11x/MLIB/bam_f16/MLIB_VMac_F16/copyright ==

== system ammclib_bam_s32k11x/MLIB/bam_f16/MLIB_VMac_F16/copyright2 ==

== system ammclib_bam_s32k11x/MLIB/bam_f16/MLIB_VMac_F16/logo ==

== system ammclib_bam_s32k11x/MLIB/bam_f32/MLIB_AbsSat_F32/copyright ==

== system ammclib_bam_s32k11x/MLIB/bam_f32/MLIB_AbsSat_F32/copyright2 ==

== system ammclib_bam_s32k11x/MLIB/bam_f32/MLIB_AbsSat_F32/logo ==

== system ammclib_bam_s32k11x/MLIB/bam_f32/MLIB_Abs_F32/copyright ==

== system ammclib_bam_s32k11x/MLIB/bam_f32/MLIB_Abs_F32/copyright2 ==

== system ammclib_bam_s32k11x/MLIB/bam_f32/MLIB_Abs_F32/logo ==

== system ammclib_bam_s32k11x/MLIB/bam_f32/MLIB_AddSat_F32/copyright ==

== system ammclib_bam_s32k11x/MLIB/bam_f32/MLIB_AddSat_F32/copyright2 ==

== system ammclib_bam_s32k11x/MLIB/bam_f32/MLIB_AddSat_F32/logo ==

== system ammclib_bam_s32k11x/MLIB/bam_f32/MLIB_Add_F32/copyright ==

== system ammclib_bam_s32k11x/MLIB/bam_f32/MLIB_Add_F32/copyright2 ==

== system ammclib_bam_s32k11x/MLIB/bam_f32/MLIB_Add_F32/logo ==

== system ammclib_bam_s32k11x/MLIB/bam_f32/MLIB_ConvertPU_F32F16/copyright ==

== system ammclib_bam_s32k11x/MLIB/bam_f32/MLIB_ConvertPU_F32F16/copyright2 ==

== system ammclib_bam_s32k11x/MLIB/bam_f32/MLIB_ConvertPU_F32F16/logo ==

== system ammclib_bam_s32k11x/MLIB/bam_f32/MLIB_Convert_F32F16/copyright ==

== system ammclib_bam_s32k11x/MLIB/bam_f32/MLIB_Convert_F32F16/copyright2 ==

== system ammclib_bam_s32k11x/MLIB/bam_f32/MLIB_Convert_F32F16/logo ==

== system ammclib_bam_s32k11x/MLIB/bam_f32/MLIB_DivSat_F32/copyright ==

== system ammclib_bam_s32k11x/MLIB/bam_f32/MLIB_DivSat_F32/copyright2 ==

== system ammclib_bam_s32k11x/MLIB/bam_f32/MLIB_DivSat_F32/logo ==

== system ammclib_bam_s32k11x/MLIB/bam_f32/MLIB_Div_F32/copyright ==

== system ammclib_bam_s32k11x/MLIB/bam_f32/MLIB_Div_F32/copyright2 ==

== system ammclib_bam_s32k11x/MLIB/bam_f32/MLIB_Div_F32/logo ==

== system ammclib_bam_s32k11x/MLIB/bam_f32/MLIB_MacSat_F32/copyright ==

== system ammclib_bam_s32k11x/MLIB/bam_f32/MLIB_MacSat_F32/copyright2 ==

== system ammclib_bam_s32k11x/MLIB/bam_f32/MLIB_MacSat_F32/logo ==

== system ammclib_bam_s32k11x/MLIB/bam_f32/MLIB_Mac_F32/copyright ==

== system ammclib_bam_s32k11x/MLIB/bam_f32/MLIB_Mac_F32/copyright2 ==

== system ammclib_bam_s32k11x/MLIB/bam_f32/MLIB_Mac_F32/logo ==

== system ammclib_bam_s32k11x/MLIB/bam_f32/MLIB_Mnac_F32/copyright ==

== system ammclib_bam_s32k11x/MLIB/bam_f32/MLIB_Mnac_F32/copyright2 ==

== system ammclib_bam_s32k11x/MLIB/bam_f32/MLIB_Mnac_F32/logo ==

== system ammclib_bam_s32k11x/MLIB/bam_f32/MLIB_Msu_F32/copyright ==

== system ammclib_bam_s32k11x/MLIB/bam_f32/MLIB_Msu_F32/copyright2 ==

== system ammclib_bam_s32k11x/MLIB/bam_f32/MLIB_Msu_F32/logo ==

== system ammclib_bam_s32k11x/MLIB/bam_f32/MLIB_MulSat_F32/copyright ==

== system ammclib_bam_s32k11x/MLIB/bam_f32/MLIB_MulSat_F32/copyright2 ==

== system ammclib_bam_s32k11x/MLIB/bam_f32/MLIB_MulSat_F32/logo ==

== system ammclib_bam_s32k11x/MLIB/bam_f32/MLIB_Mul_F32/copyright ==

== system ammclib_bam_s32k11x/MLIB/bam_f32/MLIB_Mul_F32/copyright2 ==

== system ammclib_bam_s32k11x/MLIB/bam_f32/MLIB_Mul_F32/logo ==

== system ammclib_bam_s32k11x/MLIB/bam_f32/MLIB_NegSat_F32/copyright ==

== system ammclib_bam_s32k11x/MLIB/bam_f32/MLIB_NegSat_F32/copyright2 ==

== system ammclib_bam_s32k11x/MLIB/bam_f32/MLIB_NegSat_F32/logo ==

== system ammclib_bam_s32k11x/MLIB/bam_f32/MLIB_Neg_F32/copyright ==

== system ammclib_bam_s32k11x/MLIB/bam_f32/MLIB_Neg_F32/copyright2 ==

== system ammclib_bam_s32k11x/MLIB/bam_f32/MLIB_Neg_F32/logo ==

== system ammclib_bam_s32k11x/MLIB/bam_f32/MLIB_Norm_F32/copyright ==

== system ammclib_bam_s32k11x/MLIB/bam_f32/MLIB_Norm_F32/copyright2 ==

== system ammclib_bam_s32k11x/MLIB/bam_f32/MLIB_Norm_F32/logo ==

== system ammclib_bam_s32k11x/MLIB/bam_f32/MLIB_Round_F32/copyright ==

== system ammclib_bam_s32k11x/MLIB/bam_f32/MLIB_Round_F32/copyright2 ==

== system ammclib_bam_s32k11x/MLIB/bam_f32/MLIB_Round_F32/logo ==

== system ammclib_bam_s32k11x/MLIB/bam_f32/MLIB_ShBiSat_F32/copyright ==

== system ammclib_bam_s32k11x/MLIB/bam_f32/MLIB_ShBiSat_F32/copyright2 ==

== system ammclib_bam_s32k11x/MLIB/bam_f32/MLIB_ShBiSat_F32/logo ==

== system ammclib_bam_s32k11x/MLIB/bam_f32/MLIB_ShBi_F32/copyright ==

== system ammclib_bam_s32k11x/MLIB/bam_f32/MLIB_ShBi_F32/copyright2 ==

== system ammclib_bam_s32k11x/MLIB/bam_f32/MLIB_ShBi_F32/logo ==

== system ammclib_bam_s32k11x/MLIB/bam_f32/MLIB_ShLSat_F32/copyright ==

== system ammclib_bam_s32k11x/MLIB/bam_f32/MLIB_ShLSat_F32/copyright2 ==

== system ammclib_bam_s32k11x/MLIB/bam_f32/MLIB_ShLSat_F32/logo ==

== system ammclib_bam_s32k11x/MLIB/bam_f32/MLIB_ShL_F32/copyright ==

== system ammclib_bam_s32k11x/MLIB/bam_f32/MLIB_ShL_F32/copyright2 ==

== system ammclib_bam_s32k11x/MLIB/bam_f32/MLIB_ShL_F32/logo ==

== system ammclib_bam_s32k11x/MLIB/bam_f32/MLIB_ShR_F32/copyright ==

== system ammclib_bam_s32k11x/MLIB/bam_f32/MLIB_ShR_F32/copyright2 ==

== system ammclib_bam_s32k11x/MLIB/bam_f32/MLIB_ShR_F32/logo ==

== system ammclib_bam_s32k11x/MLIB/bam_f32/MLIB_SubSat_F32/copyright ==

== system ammclib_bam_s32k11x/MLIB/bam_f32/MLIB_SubSat_F32/copyright2 ==

== system ammclib_bam_s32k11x/MLIB/bam_f32/MLIB_SubSat_F32/logo ==

== system ammclib_bam_s32k11x/MLIB/bam_f32/MLIB_Sub_F32/copyright ==

== system ammclib_bam_s32k11x/MLIB/bam_f32/MLIB_Sub_F32/copyright2 ==

== system ammclib_bam_s32k11x/MLIB/bam_f32/MLIB_Sub_F32/logo ==

== system ammclib_bam_s32k11x/MLIB/bam_f32/MLIB_VMac_F32/copyright ==

== system ammclib_bam_s32k11x/MLIB/bam_f32/MLIB_VMac_F32/copyright2 ==

== system ammclib_bam_s32k11x/MLIB/bam_f32/MLIB_VMac_F32/logo ==

== system ammclib_bam_s32k11x/MLIB/bam_f32f16f16/MLIB_MacSat_F32F16F16/copyright ==

== system ammclib_bam_s32k11x/MLIB/bam_f32f16f16/MLIB_MacSat_F32F16F16/copyright2 ==

== system ammclib_bam_s32k11x/MLIB/bam_f32f16f16/MLIB_MacSat_F32F16F16/logo ==

== system ammclib_bam_s32k11x/MLIB/bam_f32f16f16/MLIB_Mac_F32F16F16/copyright ==

== system ammclib_bam_s32k11x/MLIB/bam_f32f16f16/MLIB_Mac_F32F16F16/copyright2 ==

== system ammclib_bam_s32k11x/MLIB/bam_f32f16f16/MLIB_Mac_F32F16F16/logo ==

== system ammclib_bam_s32k11x/MLIB/bam_f32f16f16/MLIB_Mnac_F32F16F16/copyright ==

== system ammclib_bam_s32k11x/MLIB/bam_f32f16f16/MLIB_Mnac_F32F16F16/copyright2 ==

== system ammclib_bam_s32k11x/MLIB/bam_f32f16f16/MLIB_Mnac_F32F16F16/logo ==

== system ammclib_bam_s32k11x/MLIB/bam_f32f16f16/MLIB_Msu_F32F16F16/copyright ==

== system ammclib_bam_s32k11x/MLIB/bam_f32f16f16/MLIB_Msu_F32F16F16/copyright2 ==

== system ammclib_bam_s32k11x/MLIB/bam_f32f16f16/MLIB_Msu_F32F16F16/logo ==

== system ammclib_bam_s32k11x/MLIB/bam_f32f16f16/MLIB_MulSat_F32F16F16/copyright ==

== system ammclib_bam_s32k11x/MLIB/bam_f32f16f16/MLIB_MulSat_F32F16F16/copyright2 ==

== system ammclib_bam_s32k11x/MLIB/bam_f32f16f16/MLIB_MulSat_F32F16F16/logo ==

== system ammclib_bam_s32k11x/MLIB/bam_f32f16f16/MLIB_Mul_F32F16F16/copyright ==

== system ammclib_bam_s32k11x/MLIB/bam_f32f16f16/MLIB_Mul_F32F16F16/copyright2 ==

== system ammclib_bam_s32k11x/MLIB/bam_f32f16f16/MLIB_Mul_F32F16F16/logo ==

== system ammclib_bam_s32k11x/MLIB/bam_f32f16f16/MLIB_VMac_F32F16F16/copyright ==

== system ammclib_bam_s32k11x/MLIB/bam_f32f16f16/MLIB_VMac_F32F16F16/copyright2 ==

== system ammclib_bam_s32k11x/MLIB/bam_f32f16f16/MLIB_VMac_F32F16F16/logo ==
